simulink model "InvPend"  (Simulink 7.7)
settings: Solver=ode45  StartTime=0.0  StopTime=inf  RelTol=1e-3
InitFcn:
  | InvPend_Setup
libraries: vrlib x3, jMPClib x2, simulink x1
settings Model: Creator=joncur96  LastModifiedBy=jocurrie
settings OptimizationCC: InitFltsAndDblsToZero=on
settings DebuggingCC: SaveWithParameterizedLinksMsg=none  StrictBusMsg=Warning

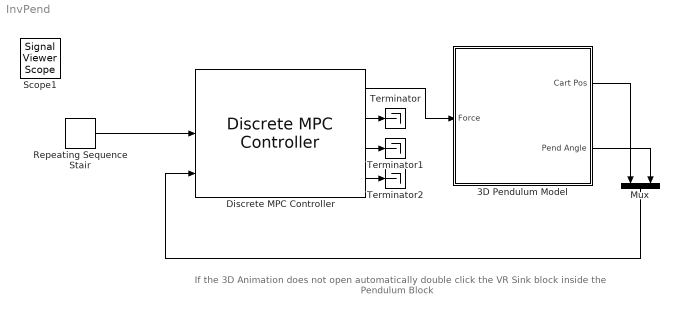
== system InvPend ==
  note: If the 3D Animation does not open automatically double click the VR Sink block inside the Pendulum Block
  3D Pendulum Model : Subsystem
      mask Display:
      | image(imread('Images/InvPendblock.png'))
      | port_label('input', 1, 'Cart Force')
      | port_label('output', 1, 'Cart Position')
      | port_label('output', 2, 'Pend Angle')
  Discrete MPC Controller : jMPClib/MPC Blocks/Discrete MPC Controller  SystemSampleTime=-1  MPC1=MPC1
  Mux : Mux  Inputs=2
  Repeating Sequence Stair : simulink/Sources/Repeating Sequence Stair  SystemSampleTime=-1  OutValues=[0 -1 2 4 1 -2.2 -4 -1 1.5 3 1]  tsamp=5  OutMin=[]  OutMax=[]  OutDataTypeStr=double  OutputDataTypeScalingMode=double  OutDataType=fixdt(0,8)  ConRadixGroup=Best Precision: Vector-wise  OutScaling=2^-12
  Terminator : Terminator
  Terminator1 : Terminator
  Terminator2 : Terminator
  Scope1 : SignalViewerScope  IOType=viewer  RefreshTime=0.035000
  wires:
  Discrete MPC Controller/1 -> 3D Pendulum Model/1(Force)
  Mux/1 -> Discrete MPC Controller/3
  3D Pendulum Model/2(Pend Angle) -> Mux/2
  3D Pendulum Model/1(Cart Pos) -> Mux/1
  Repeating Sequence Stair/1 -> Discrete MPC Controller/2
  Discrete MPC Controller/2 -> Terminator/1
  Discrete MPC Controller/3 -> Terminator1/1
  Discrete MPC Controller/4 -> Terminator2/1

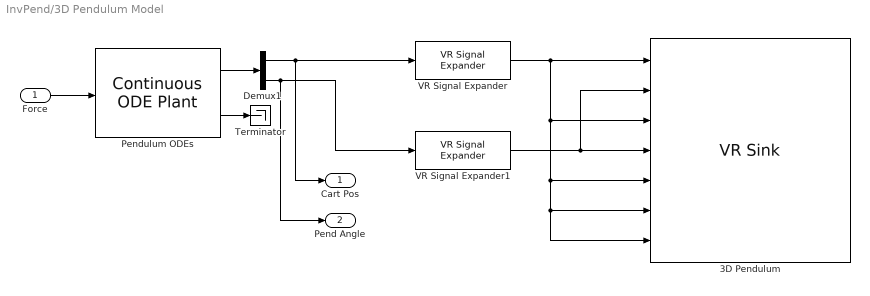
== system InvPend/3D Pendulum Model ==
  Force : Inport
  3D Pendulum : vrlib/VR Sink  SampleTime=0.1  ViewEnable=on  RemoteChange=off  RemoteView=off  FieldsWritten=Cart.translation.3.1.1.double#Pendulum.rotation.4.1.1.double#Pendulum.translation.3.1.1.double#Ball.rotation.4.1.1.double#Ball.translation.3.1.1.double#Bracket.translation.3.1.1.double#Wheels.translation.3.1.1.double  WorldFileName=InvPend.wrl  WorldDescription=Inverted Pendulum on Cart  AutoView=on  VideoDimensions=[]  FigureProperties="{'Position', 'Name', 'Viewpoint', 'CameraBound', 'CameraDirection', 'CameraPosition', 'CameraUpVector', 'ZoomFactor', 'Antialiasing', 'Headlight', 'Lighting', 'NavPanel', 'StatusBar', 'ToolBar', 'Textures', 'Transparency', 'Wireframe', 'NavZones', 'NavMode', 'NavSpeed', 'Record2DCompressMethod', 'Record2DCompressQuality', 'Record2D', 'Record2DFileName', 'Record2DFPS'; [1.6700000000000000e+002  3.3300000000000000e+002  5.7600000000000000e+002  3.8000000000000000e+002], 'Inverted Pendulum on Cart', 'Normal', 'on', [0.0000000000000000e+000  0.0000000000000000e+000 -1.0000000000000000e+000], [0.0000000000000000e+000  0.0000000000000000e+000  0.0000000000000000e+000], [0.0000000000000000e+000  1.0000000000000000e+000  0.0000000000000000e+000], [1.0000000000000000e+000], 'on', 'on', 'on', 'halfbar', 'on', 'on', 'on', 'on', 'off', 'off', 'examine', 'normal', 'auto', [7.5000000000000000e+001], 'off', '%f_anim_%n.avi', [1.5000000000000000e+001]}"
  Demux1 : Demux  Outputs=2
  Pendulum ODEs : jMPClib/MPC Blocks/Continuous ODE Plant  jNLObj=Plant
  Terminator : Terminator
  VR Signal Expander : vrlib/VR Signal Expander  SystemSampleTime=-1  outwidth=3  outidx=1
  VR Signal Expander1 : vrlib/VR Signal Expander  SystemSampleTime=-1  outwidth=4  outidx=4
  Cart Pos : Outport
  Pend Angle : Outport  Port=2
  wires:
  VR Signal Expander/1 -> 3D Pendulum/1, 3D Pendulum/3, 3D Pendulum/5, 3D Pendulum/6, 3D Pendulum/7
  VR Signal Expander1/1 -> 3D Pendulum/2, 3D Pendulum/4
  Force/1 -> Pendulum ODEs/1
  Pendulum ODEs/1 -> Demux1/1
  Demux1/1 -> VR Signal Expander/1, Cart Pos/1
  Demux1/2 -> VR Signal Expander1/1, Pend Angle/1
  Pendulum ODEs/2 -> Terminator/1
